simulink model "ExoskeletonControlModel"  (R2022b)
settings: Solver=ode3  StartTime=0.0  StopTime=inf  FixedStep=Ts  RelTol=1e-3
PreLoadFcn:
  | Ts_IO204 = 0.001;
  | 
  | if ~exist('Ts', 'var')
  | Ts = 0.001;
  | end
  | if ~exist('FPGA_Frequency', 'var')
  | FPGA_Frequency = 75000000;
  | end
  | 
  | ts_IO612 = 1e-3;
  | 
  | load('TargetReached.mat')
  | load('ActualPos_inc.mat')
model workspace (MAT data in the model file):
  DeltaData : timeseries (value not decoded)
  EC45_deg2incs = 2276
  EC60_deg2inc = 5461
  EC90_deg2incs = 7111
  Enc2rad_18bit = 2.3968e-05
  Enc2rad_19bit = 1.1984e-05
  Enc2rad_20bit = 5.9921e-06
  GiulioModel : robotics.RigidBodyTree (value not decoded)
  Giulio_Spheric_model : robotics.RigidBodyTree (value not decoded)
  Offset1_ticks = 571315
  Offset2_ticks = 590938.9928
  Offset3_ticks = 457912.8279
  Offset4_ticks = 482293.9763
  Offset5_ticks = 598735.9316
  Offset_M1 = 1.12645499896
  Offset_M2 = 4.02728553608
  Offset_M3 = 5.48587511336
  Offset_M4 = 2.03717511516
  Offset_M5 = 4.4996674016
  T1_Nm : object (value not decoded)
  T2_Nm : object (value not decoded)
  TBmodel : robotics.RigidBodyTree (value not decoded)
  Ts = 0.002
  Xg : object (value not decoded)
  Yg : object (value not decoded)
  Zg : object (value not decoded)
  a2 = 0.27
  change_variable = 0
  d1 = [0 0 0 0 0 0 0 0 0 0 0 0 ... (30001 elements, 30001x1)]
  d1_1 = 0.21074
  d2 = [0 0 0 0 0 0 0 0 0 0 0 0 ... (30001 elements, 30001x1)]
  d2_1 = 0.04864
  d3 = [0 0 0 0 0 0 0 0 0 0 0 0 ... (30001 elements, 30001x1)]
  d4 = [0 0 0 0 0 0 0 0 0 0 0 0 ... (30001 elements, 30001x1)]
  d5 = [0 0 0 0 0 0 0 0 0 0 0 0 ... (30001 elements, 30001x1)]
  d6 = [0 0 0 0 0 0 0 0 0 0 0 0 ... (30001 elements, 30001x1)]
  ee_x = -0.2852
  ee_y = -0.3683
  ee_z = -0.0386
  enc2rad_EC45 = 7.6699e-06
  enc2rad_EC90 = 2.3969e-05
  k1_Nm_ticks = 0.00923
  k2_Nm_ticks = 0.0257
  k3_Nm_ticks = 0.00692
  k4_Nm_ticks = 0.00729
  k5_Nm_ticks = 0.00641
  lower_lim_m1 = -330000
  lower_lim_m2 = -235302
  lower_lim_m3 = -132865
  lower_lim_m4 = -152732
  lower_lim_m5 = -138363
  lower_lim_m6 = -200325
  m1 = 2.441408578
  m2 = 3.750007
  m3 = 1.56250298
  m4 = 1.56250298
  m5 = 1.56250298
  m6 = 1.56250298
  n_oversampling = 8
  offset_sea_1 = 0.5547
  offset_sea_2 = 2.8595
  offset_sea_3 = 3.5058
  offset_sea_4 = 2.8586
  offset_sea_5 = 2.8736
  params : AKSIM (value not decoded)
  pos_th_neg = -180000
  pos_th_pos = 180000
  q1 = -1819347
  q2 = -196752
  q3 = -596465
  q4 = -556807
  q5 = -573932
  q6 = -489063
  sine = [0 0.187999937334 0.751998997352 1.69199492401 3.0079839574 4.6999608335 6.76791878442 9.21184953835 12.0317433196 15.2275888485 18.7993733417 22.7470825122 ... (12501 elements, 12501x1)]
  start : object (value not decoded)
  switch_admittance = 1
  t1 : object (value not decoded)
  t2 : object (value not decoded)
  torsionalStiffnes_M1 = 384.88
  torsionalStiffnes_M2 = 1500
  torsionalStiffnes_M3 = 901.97
  torsionalStiffnes_M4 = 950.86
  torsionalStiffnes_M5 = 930
  torsionalStiffnes_M6 = 914
  upper_lim_m1 = 340000
  upper_lim_m2 = 95467
  upper_lim_m3 = 164951
  upper_lim_m4 = 210607
  upper_lim_m5 = 252595
  upper_lim_m6 = 96694
  vel_th_neg = -100
  vel_th_pos = 100
  x = 0
undefined symbols (not defined in the file): C, DiscIntNeverNeededParam
libraries: canmsglib x285, speedgoatlib_IO614 x245, simulink x26, slrealtimeloglib x9, simulink_extras x6, robotmaniplib x6
(part 3 of 13)

== system ExoskeletonControlModel/DataProcessing/Working_Chart/GoHome.GoHome_M4.ST3_send_target_pos_M4 ==
  note: MOTOR 1 - TARGET POSITION
  Action Port : ActionPort
      settings: CopyFcn=Stateflow.SLINSF.SimulinkMan.removeBlockPreDeleteFcn  PreDeleteFcn=Stateflow.SLINSF.SimulinkMan.unsafePredeleteFcn
  receive_PDO3_m1 : Subsystem
  target_position_m1 : Constant  Value=0
  wires:
  target_position_m1/1 -> receive_PDO3_m1/1(target_pos)

== system ExoskeletonControlModel/DataProcessing/Working_Chart/GoHome.GoHome_M4.ST4_Abs_ref_start_immediatly_M4 ==
  note: MOTOR 1 - CONTROLWORD
  Action Port : ActionPort
      settings: CopyFcn=Stateflow.SLINSF.SimulinkMan.removeBlockPreDeleteFcn  PreDeleteFcn=Stateflow.SLINSF.SimulinkMan.unsafePredeleteFcn
  controlword_m1 : Constant  Value=63
  receive_PDO1_m1 : Subsystem
  wires:
  controlword_m1/1 -> receive_PDO1_m1/1(controlword)

== system ExoskeletonControlModel/DataProcessing/Working_Chart/GoHome.GoHome_M5.ST1_set_PPM_M5 ==
  note: MOTOR 1 - MODE & INTERPOLATION TIME PERIOD
  Action Port : ActionPort
      settings: CopyFcn=Stateflow.SLINSF.SimulinkMan.removeBlockPreDeleteFcn  PreDeleteFcn=Stateflow.SLINSF.SimulinkMan.unsafePredeleteFcn
  Bus Creator3 : BusCreator  Inputs=2
  interpolation_period_m1 : Constant  Value=10
  mode_m1 : Constant
  receive_PDO2_m1 : Subsystem
  wires:
  Bus Creator3/1 -> receive_PDO2_m1/1(mode)
  mode_m1/1 -> Bus Creator3/1  "mode_m1"
  interpolation_period_m1/1 -> Bus Creator3/2  "interpolation_period_m1"

== system ExoskeletonControlModel/DataProcessing/Working_Chart/GoHome.GoHome_M5.ST2_Switch_on_Enable_M5 ==
  note: MOTOR 1 - CONTROLWORD
  Action Port : ActionPort
      settings: CopyFcn=Stateflow.SLINSF.SimulinkMan.removeBlockPreDeleteFcn  PreDeleteFcn=Stateflow.SLINSF.SimulinkMan.unsafePredeleteFcn
  controlword_m1 : Constant  Value=15
  receive_PDO1_m1 : Subsystem
  wires:
  controlword_m1/1 -> receive_PDO1_m1/1(controlword)

== system ExoskeletonControlModel/DataProcessing/Working_Chart/GoHome.GoHome_M5.ST3_send_target_pos_M5 ==
  note: MOTOR 1 - TARGET POSITION
  Action Port : ActionPort
      settings: CopyFcn=Stateflow.SLINSF.SimulinkMan.removeBlockPreDeleteFcn  PreDeleteFcn=Stateflow.SLINSF.SimulinkMan.unsafePredeleteFcn
  receive_PDO3_m1 : Subsystem
  target_position_m1 : Constant  Value=0
  wires:
  target_position_m1/1 -> receive_PDO3_m1/1(target_pos)

== system ExoskeletonControlModel/DataProcessing/Working_Chart/GoHome.GoHome_M5.ST4_Abs_ref_start_immediatly_M5 ==
  note: MOTOR 1 - CONTROLWORD
  Action Port : ActionPort
      settings: CopyFcn=Stateflow.SLINSF.SimulinkMan.removeBlockPreDeleteFcn  PreDeleteFcn=Stateflow.SLINSF.SimulinkMan.unsafePredeleteFcn
  controlword_m1 : Constant  Value=63
  receive_PDO1_m1 : Subsystem
  wires:
  controlword_m1/1 -> receive_PDO1_m1/1(controlword)

== system ExoskeletonControlModel/DataProcessing/Working_Chart/GoHome.GoHome_M6.ST1_set_PPM_M6 ==
  note: MOTOR 1 - MODE & INTERPOLATION TIME PERIOD
  Action Port : ActionPort
      settings: CopyFcn=Stateflow.SLINSF.SimulinkMan.removeBlockPreDeleteFcn  PreDeleteFcn=Stateflow.SLINSF.SimulinkMan.unsafePredeleteFcn
  Bus Creator3 : BusCreator  Inputs=2
  interpolation_period_m1 : Constant  Value=10
  mode_m1 : Constant
  receive_PDO2_m1 : Subsystem
  wires:
  Bus Creator3/1 -> receive_PDO2_m1/1(mode)
  mode_m1/1 -> Bus Creator3/1  "mode_m1"
  interpolation_period_m1/1 -> Bus Creator3/2  "interpolation_period_m1"

== system ExoskeletonControlModel/DataProcessing/Working_Chart/GoHome.GoHome_M6.ST2_Switch_on_Enable_M6 ==
  note: MOTOR 1 - CONTROLWORD
  Action Port : ActionPort
      settings: CopyFcn=Stateflow.SLINSF.SimulinkMan.removeBlockPreDeleteFcn  PreDeleteFcn=Stateflow.SLINSF.SimulinkMan.unsafePredeleteFcn
  controlword_m1 : Constant  Value=15
  receive_PDO1_m1 : Subsystem
  wires:
  controlword_m1/1 -> receive_PDO1_m1/1(controlword)

== system ExoskeletonControlModel/DataProcessing/Working_Chart/GoHome.GoHome_M6.ST3_send_target_pos_M6 ==
  note: MOTOR 1 - TARGET POSITION
  Action Port : ActionPort
      settings: CopyFcn=Stateflow.SLINSF.SimulinkMan.removeBlockPreDeleteFcn  PreDeleteFcn=Stateflow.SLINSF.SimulinkMan.unsafePredeleteFcn
  receive_PDO3_m1 : Subsystem
  target_position_m1 : Constant  Value=0
  wires:
  target_position_m1/1 -> receive_PDO3_m1/1(target_pos)

== system ExoskeletonControlModel/DataProcessing/Working_Chart/GoHome.GoHome_M6.ST4_Abs_ref_start_immediatly_M6 ==
  note: MOTOR 1 - CONTROLWORD
  Action Port : ActionPort
      settings: CopyFcn=Stateflow.SLINSF.SimulinkMan.removeBlockPreDeleteFcn  PreDeleteFcn=Stateflow.SLINSF.SimulinkMan.unsafePredeleteFcn
  controlword_m1 : Constant  Value=63
  receive_PDO1_m1 : Subsystem
  wires:
  controlword_m1/1 -> receive_PDO1_m1/1(controlword)

== system ExoskeletonControlModel/DataProcessing/Working_Chart/Transparency.Block_not_recorded_joints.ST1_set_CSP_M1 ==
  note: MOTOR 1 - MODE & INTERPOLATION TIME PERIOD
  Action Port : ActionPort
      settings: CopyFcn=Stateflow.SLINSF.SimulinkMan.removeBlockPreDeleteFcn  PreDeleteFcn=Stateflow.SLINSF.SimulinkMan.unsafePredeleteFcn
  Bus Creator3 : BusCreator  Inputs=2
  interpolation_period_m1 : Constant  Value=20
  mode_m1 : Constant  Value=8
  receive_PDO2_m1 : Subsystem
  wires:
  Bus Creator3/1 -> receive_PDO2_m1/1(mode)
  mode_m1/1 -> Bus Creator3/1  "mode_m1"
  interpolation_period_m1/1 -> Bus Creator3/2  "interpolation_period_m1"

== system ExoskeletonControlModel/DataProcessing/Working_Chart/Transparency.Block_not_recorded_joints.ST1_set_CSP_M6 ==
  note: MOTOR 1 - MODE & INTERPOLATION TIME PERIOD
  Action Port : ActionPort
      settings: CopyFcn=Stateflow.SLINSF.SimulinkMan.removeBlockPreDeleteFcn  PreDeleteFcn=Stateflow.SLINSF.SimulinkMan.unsafePredeleteFcn
  Bus Creator3 : BusCreator  Inputs=2
  interpolation_period_m1 : Constant  Value=20
  mode_m1 : Constant  Value=8
  receive_PDO2_m1 : Subsystem
  wires:
  Bus Creator3/1 -> receive_PDO2_m1/1(mode)
  mode_m1/1 -> Bus Creator3/1  "mode_m1"
  interpolation_period_m1/1 -> Bus Creator3/2  "interpolation_period_m1"

== system ExoskeletonControlModel/DataProcessing/Working_Chart/Transparency.GoToExerciseHome.GoHome_M1.ST1_set_PPM_M1 ==
  note: MOTOR 1 - MODE & INTERPOLATION TIME PERIOD
  Action Port : ActionPort
      settings: CopyFcn=Stateflow.SLINSF.SimulinkMan.removeBlockPreDeleteFcn  PreDeleteFcn=Stateflow.SLINSF.SimulinkMan.unsafePredeleteFcn
  Bus Creator3 : BusCreator  Inputs=2
  interpolation_period_m1 : Constant  Value=10
  mode_m1 : Constant
  receive_PDO2_m1 : Subsystem
  wires:
  Bus Creator3/1 -> receive_PDO2_m1/1(mode)
  mode_m1/1 -> Bus Creator3/1  "mode_m1"
  interpolation_period_m1/1 -> Bus Creator3/2  "interpolation_period_m1"

== system ExoskeletonControlModel/DataProcessing/Working_Chart/Transparency.GoToExerciseHome.GoHome_M1.ST2_Switch_on_Enable_M1 ==
  note: MOTOR 1 - CONTROLWORD
  Action Port : ActionPort
      settings: CopyFcn=Stateflow.SLINSF.SimulinkMan.removeBlockPreDeleteFcn  PreDeleteFcn=Stateflow.SLINSF.SimulinkMan.unsafePredeleteFcn
  controlword_m1 : Constant  Value=15
  receive_PDO1_m1 : Subsystem
  wires:
  controlword_m1/1 -> receive_PDO1_m1/1(controlword)

== system ExoskeletonControlModel/DataProcessing/Working_Chart/Transparency.GoToExerciseHome.GoHome_M1.ST3_send_target_pos_M1 ==
  note: MOTOR 1 - TARGET POSITION
  Action Port : ActionPort
      settings: CopyFcn=Stateflow.SLINSF.SimulinkMan.removeBlockPreDeleteFcn  PreDeleteFcn=Stateflow.SLINSF.SimulinkMan.unsafePredeleteFcn
  receive_PDO3_m1 : Subsystem
  target_position_m1 : Constant  Value=0
  wires:
  target_position_m1/1 -> receive_PDO3_m1/1(target_pos)

== system ExoskeletonControlModel/DataProcessing/Working_Chart/Transparency.GoToExerciseHome.GoHome_M1.ST4_Abs_ref_start_immediatly_M1 ==
  note: MOTOR 1 - CONTROLWORD
  Action Port : ActionPort
      settings: CopyFcn=Stateflow.SLINSF.SimulinkMan.removeBlockPreDeleteFcn  PreDeleteFcn=Stateflow.SLINSF.SimulinkMan.unsafePredeleteFcn
  controlword_m1 : Constant  Value=63
  receive_PDO1_m1 : Subsystem
  wires:
  controlword_m1/1 -> receive_PDO1_m1/1(controlword)

== system ExoskeletonControlModel/DataProcessing/Working_Chart/Transparency.GoToExerciseHome.GoHome_M2.ST1_set_PPM_M2 ==
  note: MOTOR 1 - MODE & INTERPOLATION TIME PERIOD
  Action Port : ActionPort
      settings: CopyFcn=Stateflow.SLINSF.SimulinkMan.removeBlockPreDeleteFcn  PreDeleteFcn=Stateflow.SLINSF.SimulinkMan.unsafePredeleteFcn
  Bus Creator3 : BusCreator  Inputs=2
  interpolation_period_m1 : Constant  Value=10
  mode_m1 : Constant
  receive_PDO2_m1 : Subsystem
  wires:
  Bus Creator3/1 -> receive_PDO2_m1/1(mode)
  mode_m1/1 -> Bus Creator3/1  "mode_m1"
  interpolation_period_m1/1 -> Bus Creator3/2  "interpolation_period_m1"

== system ExoskeletonControlModel/DataProcessing/Working_Chart/Transparency.GoToExerciseHome.GoHome_M2.ST2_Switch_on_Enable_M2 ==
  note: MOTOR 1 - CONTROLWORD
  Action Port : ActionPort
      settings: CopyFcn=Stateflow.SLINSF.SimulinkMan.removeBlockPreDeleteFcn  PreDeleteFcn=Stateflow.SLINSF.SimulinkMan.unsafePredeleteFcn
  controlword_m1 : Constant  Value=15
  receive_PDO1_m1 : Subsystem
  wires:
  controlword_m1/1 -> receive_PDO1_m1/1(controlword)

== system ExoskeletonControlModel/DataProcessing/Working_Chart/Transparency.GoToExerciseHome.GoHome_M2.ST3_send_target_pos_M2 ==
  note: MOTOR 1 - TARGET POSITION
  Action Port : ActionPort
      settings: CopyFcn=Stateflow.SLINSF.SimulinkMan.removeBlockPreDeleteFcn  PreDeleteFcn=Stateflow.SLINSF.SimulinkMan.unsafePredeleteFcn
  receive_PDO3_m1 : Subsystem
  target_position_m1 : Constant  Value=0
  wires:
  target_position_m1/1 -> receive_PDO3_m1/1(target_pos)

== system ExoskeletonControlModel/DataProcessing/Working_Chart/Transparency.GoToExerciseHome.GoHome_M2.ST4_Abs_ref_start_immediatly_M2 ==
  note: MOTOR 1 - CONTROLWORD
  Action Port : ActionPort
      settings: CopyFcn=Stateflow.SLINSF.SimulinkMan.removeBlockPreDeleteFcn  PreDeleteFcn=Stateflow.SLINSF.SimulinkMan.unsafePredeleteFcn
  controlword_m1 : Constant  Value=63
  receive_PDO1_m1 : Subsystem
  wires:
  controlword_m1/1 -> receive_PDO1_m1/1(controlword)

== system ExoskeletonControlModel/DataProcessing/Working_Chart/Transparency.GoToExerciseHome.GoHome_M3.ST1_set_PPM_M3 ==
  note: MOTOR 1 - MODE & INTERPOLATION TIME PERIOD
  Action Port : ActionPort
      settings: CopyFcn=Stateflow.SLINSF.SimulinkMan.removeBlockPreDeleteFcn  PreDeleteFcn=Stateflow.SLINSF.SimulinkMan.unsafePredeleteFcn
  Bus Creator3 : BusCreator  Inputs=2
  interpolation_period_m1 : Constant  Value=10
  mode_m1 : Constant
  receive_PDO2_m1 : Subsystem
  wires:
  Bus Creator3/1 -> receive_PDO2_m1/1(mode)
  mode_m1/1 -> Bus Creator3/1  "mode_m1"
  interpolation_period_m1/1 -> Bus Creator3/2  "interpolation_period_m1"

== system ExoskeletonControlModel/DataProcessing/Working_Chart/Transparency.GoToExerciseHome.GoHome_M3.ST2_Switch_on_Enable_M3 ==
  note: MOTOR 1 - CONTROLWORD
  Action Port : ActionPort
      settings: CopyFcn=Stateflow.SLINSF.SimulinkMan.removeBlockPreDeleteFcn  PreDeleteFcn=Stateflow.SLINSF.SimulinkMan.unsafePredeleteFcn
  controlword_m1 : Constant  Value=15
  receive_PDO1_m1 : Subsystem
  wires:
  controlword_m1/1 -> receive_PDO1_m1/1(controlword)

== system ExoskeletonControlModel/DataProcessing/Working_Chart/Transparency.GoToExerciseHome.GoHome_M3.ST3_send_target_pos_M3 ==
  note: MOTOR 3 - TARGET POSITION
  Action Port : ActionPort
      settings: CopyFcn=Stateflow.SLINSF.SimulinkMan.removeBlockPreDeleteFcn  PreDeleteFcn=Stateflow.SLINSF.SimulinkMan.unsafePredeleteFcn
  receive_PDO3_m1 : Subsystem
  target_position_m1 : Constant  Value=50153
  wires:
  target_position_m1/1 -> receive_PDO3_m1/1(target_pos)

== system ExoskeletonControlModel/DataProcessing/Working_Chart/Transparency.GoToExerciseHome.GoHome_M3.ST4_Abs_ref_start_immediatly_M3 ==
  note: MOTOR 1 - CONTROLWORD
  Action Port : ActionPort
      settings: CopyFcn=Stateflow.SLINSF.SimulinkMan.removeBlockPreDeleteFcn  PreDeleteFcn=Stateflow.SLINSF.SimulinkMan.unsafePredeleteFcn
  controlword_m1 : Constant  Value=63
  receive_PDO1_m1 : Subsystem
  wires:
  controlword_m1/1 -> receive_PDO1_m1/1(controlword)

== system ExoskeletonControlModel/DataProcessing/Working_Chart/Transparency.GoToExerciseHome.GoHome_M4.ST1_set_PPM_M4 ==
  note: MOTOR 1 - MODE & INTERPOLATION TIME PERIOD
  Action Port : ActionPort
      settings: CopyFcn=Stateflow.SLINSF.SimulinkMan.removeBlockPreDeleteFcn  PreDeleteFcn=Stateflow.SLINSF.SimulinkMan.unsafePredeleteFcn
  Bus Creator3 : BusCreator  Inputs=2
  interpolation_period_m1 : Constant  Value=10
  mode_m1 : Constant
  receive_PDO2_m1 : Subsystem
  wires:
  Bus Creator3/1 -> receive_PDO2_m1/1(mode)
  mode_m1/1 -> Bus Creator3/1  "mode_m1"
  interpolation_period_m1/1 -> Bus Creator3/2  "interpolation_period_m1"

== system ExoskeletonControlModel/DataProcessing/Working_Chart/Transparency.GoToExerciseHome.GoHome_M4.ST2_Switch_on_Enable_M4 ==
  note: MOTOR 1 - CONTROLWORD
  Action Port : ActionPort
      settings: CopyFcn=Stateflow.SLINSF.SimulinkMan.removeBlockPreDeleteFcn  PreDeleteFcn=Stateflow.SLINSF.SimulinkMan.unsafePredeleteFcn
  controlword_m1 : Constant  Value=15
  receive_PDO1_m1 : Subsystem
  wires:
  controlword_m1/1 -> receive_PDO1_m1/1(controlword)

== system ExoskeletonControlModel/DataProcessing/Working_Chart/Transparency.GoToExerciseHome.GoHome_M4.ST3_send_target_pos_M4 ==
  note: MOTOR 4 - TARGET POSITION
  Action Port : ActionPort
      settings: CopyFcn=Stateflow.SLINSF.SimulinkMan.removeBlockPreDeleteFcn  PreDeleteFcn=Stateflow.SLINSF.SimulinkMan.unsafePredeleteFcn
  receive_PDO3_m1 : Subsystem
  target_position_m1 : Constant  Value=-22699
  wires:
  target_position_m1/1 -> receive_PDO3_m1/1(target_pos)

== system ExoskeletonControlModel/DataProcessing/Working_Chart/Transparency.GoToExerciseHome.GoHome_M4.ST3_send_target_pos_M4_abd ==
  note: MOTOR 4 - TARGET POSITION
  Action Port : ActionPort
      settings: CopyFcn=Stateflow.SLINSF.SimulinkMan.removeBlockPreDeleteFcn  PreDeleteFcn=Stateflow.SLINSF.SimulinkMan.unsafePredeleteFcn
  receive_PDO3_m1 : Subsystem
  target_position_m1 : Constant  Value=-90979
  wires:
  target_position_m1/1 -> receive_PDO3_m1/1(target_pos)

== system ExoskeletonControlModel/DataProcessing/Working_Chart/Transparency.GoToExerciseHome.GoHome_M4.ST4_Abs_ref_start_immediatly_M4 ==
  note: MOTOR 1 - CONTROLWORD
  Action Port : ActionPort
      settings: CopyFcn=Stateflow.SLINSF.SimulinkMan.removeBlockPreDeleteFcn  PreDeleteFcn=Stateflow.SLINSF.SimulinkMan.unsafePredeleteFcn
  controlword_m1 : Constant  Value=63
  receive_PDO1_m1 : Subsystem
  wires:
  controlword_m1/1 -> receive_PDO1_m1/1(controlword)

== system ExoskeletonControlModel/DataProcessing/Working_Chart/Transparency.GoToExerciseHome.GoHome_M5.ST1_set_PPM_M5 ==
  note: MOTOR 1 - MODE & INTERPOLATION TIME PERIOD
  Action Port : ActionPort
      settings: CopyFcn=Stateflow.SLINSF.SimulinkMan.removeBlockPreDeleteFcn  PreDeleteFcn=Stateflow.SLINSF.SimulinkMan.unsafePredeleteFcn
  Bus Creator3 : BusCreator  Inputs=2
  interpolation_period_m1 : Constant  Value=10
  mode_m1 : Constant
  receive_PDO2_m1 : Subsystem
  wires:
  Bus Creator3/1 -> receive_PDO2_m1/1(mode)
  mode_m1/1 -> Bus Creator3/1  "mode_m1"
  interpolation_period_m1/1 -> Bus Creator3/2  "interpolation_period_m1"

== system ExoskeletonControlModel/DataProcessing/Working_Chart/Transparency.GoToExerciseHome.GoHome_M5.ST2_Switch_on_Enable_M5 ==
  note: MOTOR 1 - CONTROLWORD
  Action Port : ActionPort
      settings: CopyFcn=Stateflow.SLINSF.SimulinkMan.removeBlockPreDeleteFcn  PreDeleteFcn=Stateflow.SLINSF.SimulinkMan.unsafePredeleteFcn
  controlword_m1 : Constant  Value=15
  receive_PDO1_m1 : Subsystem
  wires:
  controlword_m1/1 -> receive_PDO1_m1/1(controlword)

== system ExoskeletonControlModel/DataProcessing/Working_Chart/Transparency.GoToExerciseHome.GoHome_M5.ST3_send_target_pos_M5 ==
  note: MOTOR 5 - TARGET POSITION
  Action Port : ActionPort
      settings: CopyFcn=Stateflow.SLINSF.SimulinkMan.removeBlockPreDeleteFcn  PreDeleteFcn=Stateflow.SLINSF.SimulinkMan.unsafePredeleteFcn
  receive_PDO3_m1 : Subsystem
  target_position_m1 : Constant  Value=-9784
  wires:
  target_position_m1/1 -> receive_PDO3_m1/1(target_pos)

== system ExoskeletonControlModel/DataProcessing/Working_Chart/Transparency.GoToExerciseHome.GoHome_M5.ST4_Abs_ref_start_immediatly_M5 ==
  note: MOTOR 1 - CONTROLWORD
  Action Port : ActionPort
      settings: CopyFcn=Stateflow.SLINSF.SimulinkMan.removeBlockPreDeleteFcn  PreDeleteFcn=Stateflow.SLINSF.SimulinkMan.unsafePredeleteFcn
  controlword_m1 : Constant  Value=63
  receive_PDO1_m1 : Subsystem
  wires:
  controlword_m1/1 -> receive_PDO1_m1/1(controlword)

== system ExoskeletonControlModel/DataProcessing/Working_Chart/Transparency.GoToExerciseHome.GoHome_M6.ST1_set_PPM_M6 ==
  note: MOTOR 1 - MODE & INTERPOLATION TIME PERIOD
  Action Port : ActionPort
      settings: CopyFcn=Stateflow.SLINSF.SimulinkMan.removeBlockPreDeleteFcn  PreDeleteFcn=Stateflow.SLINSF.SimulinkMan.unsafePredeleteFcn
  Bus Creator3 : BusCreator  Inputs=2
  interpolation_period_m1 : Constant  Value=10
  mode_m1 : Constant
  receive_PDO2_m1 : Subsystem
  wires:
  Bus Creator3/1 -> receive_PDO2_m1/1(mode)
  mode_m1/1 -> Bus Creator3/1  "mode_m1"
  interpolation_period_m1/1 -> Bus Creator3/2  "interpolation_period_m1"

== system ExoskeletonControlModel/DataProcessing/Working_Chart/Transparency.GoToExerciseHome.GoHome_M6.ST2_Switch_on_Enable_M6 ==
  note: MOTOR 1 - CONTROLWORD
  Action Port : ActionPort
      settings: CopyFcn=Stateflow.SLINSF.SimulinkMan.removeBlockPreDeleteFcn  PreDeleteFcn=Stateflow.SLINSF.SimulinkMan.unsafePredeleteFcn
  controlword_m1 : Constant  Value=15
  receive_PDO1_m1 : Subsystem
  wires:
  controlword_m1/1 -> receive_PDO1_m1/1(controlword)

== system ExoskeletonControlModel/DataProcessing/Working_Chart/Transparency.GoToExerciseHome.GoHome_M6.ST3_send_target_pos_M6 ==
  note: MOTOR 1 - TARGET POSITION
  Action Port : ActionPort
      settings: CopyFcn=Stateflow.SLINSF.SimulinkMan.removeBlockPreDeleteFcn  PreDeleteFcn=Stateflow.SLINSF.SimulinkMan.unsafePredeleteFcn
  receive_PDO3_m1 : Subsystem
  target_position_m1 : Constant  Value=-165590
  wires:
  target_position_m1/1 -> receive_PDO3_m1/1(target_pos)

== system ExoskeletonControlModel/DataProcessing/Working_Chart/Transparency.GoToExerciseHome.GoHome_M6.ST4_Abs_ref_start_immediatly_M6 ==
  note: MOTOR 1 - CONTROLWORD
  Action Port : ActionPort
      settings: CopyFcn=Stateflow.SLINSF.SimulinkMan.removeBlockPreDeleteFcn  PreDeleteFcn=Stateflow.SLINSF.SimulinkMan.unsafePredeleteFcn
  controlword_m1 : Constant  Value=63
  receive_PDO1_m1 : Subsystem
  wires:
  controlword_m1/1 -> receive_PDO1_m1/1(controlword)

== system ExoskeletonControlModel/DataProcessing/Working_Chart/Transparency.ImpedanceMode.ShoulderFlexion.ST1_set_CSP_M3 ==
  note: MOTOR 1 - MODE & INTERPOLATION TIME PERIOD
  Action Port : ActionPort
      settings: CopyFcn=Stateflow.SLINSF.SimulinkMan.removeBlockPreDeleteFcn  PreDeleteFcn=Stateflow.SLINSF.SimulinkMan.unsafePredeleteFcn
  Bus Creator3 : BusCreator  Inputs=2
  interpolation_period_m1 : Constant  Value=10
  mode_m1 : Constant  Value=8
  receive_PDO2_m1 : Subsystem
  wires:
  Bus Creator3/1 -> receive_PDO2_m1/1(mode)
  mode_m1/1 -> Bus Creator3/1  "mode_m1"
  interpolation_period_m1/1 -> Bus Creator3/2  "interpolation_period_m1"

== system ExoskeletonControlModel/DataProcessing/Working_Chart/Transparency.ImpedanceMode.ShoulderFlexion.ST1_set_CSP_M4 ==
  note: MOTOR 1 - MODE & INTERPOLATION TIME PERIOD
  Action Port : ActionPort
      settings: CopyFcn=Stateflow.SLINSF.SimulinkMan.removeBlockPreDeleteFcn  PreDeleteFcn=Stateflow.SLINSF.SimulinkMan.unsafePredeleteFcn
  Bus Creator3 : BusCreator  Inputs=2
  interpolation_period_m1 : Constant  Value=10
  mode_m1 : Constant  Value=8
  receive_PDO2_m1 : Subsystem
  wires:
  Bus Creator3/1 -> receive_PDO2_m1/1(mode)
  mode_m1/1 -> Bus Creator3/1  "mode_m1"
  interpolation_period_m1/1 -> Bus Creator3/2  "interpolation_period_m1"

== system ExoskeletonControlModel/DataProcessing/Working_Chart/Transparency.ImpedanceMode.ShoulderFlexion.ST1_set_CSP_M6 ==
  note: MOTOR 1 - MODE & INTERPOLATION TIME PERIOD
  Action Port : ActionPort
      settings: CopyFcn=Stateflow.SLINSF.SimulinkMan.removeBlockPreDeleteFcn  PreDeleteFcn=Stateflow.SLINSF.SimulinkMan.unsafePredeleteFcn
  Bus Creator3 : BusCreator  Inputs=2
  interpolation_period_m1 : Constant  Value=10
  mode_m1 : Constant  Value=8
  receive_PDO2_m1 : Subsystem
  wires:
  Bus Creator3/1 -> receive_PDO2_m1/1(mode)
  mode_m1/1 -> Bus Creator3/1  "mode_m1"
  interpolation_period_m1/1 -> Bus Creator3/2  "interpolation_period_m1"

== system ExoskeletonControlModel/DataProcessing/Working_Chart/Transparency.ResetState ==
  Action Port : ActionPort
      settings: CopyFcn=Stateflow.SLINSF.SimulinkMan.removeBlockPreDeleteFcn  PreDeleteFcn=Stateflow.SLINSF.SimulinkMan.unsafePredeleteFcn
  Constant{,1..17} (18 alike) : Constant  Value=0
  Data Store Write : DataStoreWrite  DataStoreName=Start_m1  IndexOptions=Index vector (dialog)  Indices=1  OutputSizes=1
  Data Store Write1 : DataStoreWrite  DataStoreName=Start_m3  IndexOptions=Index vector (dialog)  Indices=1  OutputSizes=1
  Data Store Write10 : DataStoreWrite  DataStoreName=Spring_m5  IndexOptions=Index vector (dialog)  Indices=1  OutputSizes=1
  Data Store Write11 : DataStoreWrite  DataStoreName=Spring_m6  IndexOptions=Index vector (dialog)  Indices=1  OutputSizes=1
  Data Store Write12 : DataStoreWrite  DataStoreName=Damper_m5  IndexOptions=Index vector (dialog)  Indices=1  OutputSizes=1
  Data Store Write13 : DataStoreWrite  DataStoreName=Damper_m6  IndexOptions=Index vector (dialog)  Indices=1  OutputSizes=1
  Data Store Write14 : DataStoreWrite  DataStoreName=Damper_m1  IndexOptions=Index vector (dialog)  Indices=1  OutputSizes=1
  Data Store Write15 : DataStoreWrite  DataStoreName=Damper_m3  IndexOptions=Index vector (dialog)  Indices=1  OutputSizes=1
  Data Store Write16 : DataStoreWrite  DataStoreName=Damper_m2  IndexOptions=Index vector (dialog)  Indices=1  OutputSizes=1
  Data Store Write17 : DataStoreWrite  DataStoreName=Damper_m4  IndexOptions=Index vector (dialog)  Indices=1  OutputSizes=1
  Data Store Write2 : DataStoreWrite  DataStoreName=Start_m2  IndexOptions=Index vector (dialog)  Indices=1  OutputSizes=1
  Data Store Write3 : DataStoreWrite  DataStoreName=Start_m4  IndexOptions=Index vector (dialog)  Indices=1  OutputSizes=1
  Data Store Write4 : DataStoreWrite  DataStoreName=Start_m5  IndexOptions=Index vector (dialog)  Indices=1  OutputSizes=1
  Data Store Write5 : DataStoreWrite  DataStoreName=Start_m6  IndexOptions=Index vector (dialog)  Indices=1  OutputSizes=1
  Data Store Write6 : DataStoreWrite  DataStoreName=Spring_m1  IndexOptions=Index vector (dialog)  Indices=1  OutputSizes=1
  Data Store Write7 : DataStoreWrite  DataStoreName=Spring_m3  IndexOptions=Index vector (dialog)  Indices=1  OutputSizes=1
  Data Store Write8 : DataStoreWrite  DataStoreName=Spring_m2  IndexOptions=Index vector (dialog)  Indices=1  OutputSizes=1
  Data Store Write9 : DataStoreWrite  DataStoreName=Spring_m4  IndexOptions=Index vector (dialog)  Indices=1  OutputSizes=1
  wires:
  Constant/1 -> Data Store Write/1
  Constant1/1 -> Data Store Write1/1
  Constant2/1 -> Data Store Write2/1
  Constant3/1 -> Data Store Write3/1
  Constant4/1 -> Data Store Write4/1
  Constant5/1 -> Data Store Write5/1
  Constant6/1 -> Data Store Write6/1
  Constant11/1 -> Data Store Write11/1
  Constant8/1 -> Data Store Write8/1
  Constant7/1 -> Data Store Write7/1
  Constant9/1 -> Data Store Write9/1
  Constant10/1 -> Data Store Write10/1
  Constant17/1 -> Data Store Write17/1
  Constant13/1 -> Data Store Write13/1
  Constant12/1 -> Data Store Write12/1
  Constant14/1 -> Data Store Write14/1
  Constant16/1 -> Data Store Write16/1
  Constant15/1 -> Data Store Write15/1

== system ExoskeletonControlModel/DataProcessing/Working_Chart/Transparency.SET_MODE.ST1_set_CSP_M2 ==
  note: MOTOR 1 - MODE & INTERPOLATION TIME PERIOD
  Action Port : ActionPort
      settings: CopyFcn=Stateflow.SLINSF.SimulinkMan.removeBlockPreDeleteFcn  PreDeleteFcn=Stateflow.SLINSF.SimulinkMan.unsafePredeleteFcn
  Bus Creator3 : BusCreator  Inputs=2
  interpolation_period_m1 : Constant  Value=10
  mode_m1 : Constant  Value=8
  receive_PDO2_m1 : Subsystem
  wires:
  Bus Creator3/1 -> receive_PDO2_m1/1(mode)
  mode_m1/1 -> Bus Creator3/1  "mode_m1"
  interpolation_period_m1/1 -> Bus Creator3/2  "interpolation_period_m1"

== system ExoskeletonControlModel/DataProcessing/Working_Chart/Transparency.SET_MODE.ST1_set_CST_M1 ==
  note: MOTOR 1 - MODE & INTERPOLATION TIME PERIOD
  Action Port : ActionPort
      settings: CopyFcn=Stateflow.SLINSF.SimulinkMan.removeBlockPreDeleteFcn  PreDeleteFcn=Stateflow.SLINSF.SimulinkMan.unsafePredeleteFcn
  Bus Creator3 : BusCreator  Inputs=2
  interpolation_period_m1 : Constant  Value=20
  mode_m1 : Constant  Value=10
  receive_PDO2_m1 : Subsystem
  wires:
  Bus Creator3/1 -> receive_PDO2_m1/1(mode)
  mode_m1/1 -> Bus Creator3/1  "mode_m1"
  interpolation_period_m1/1 -> Bus Creator3/2  "interpolation_period_m1"

== system ExoskeletonControlModel/DataProcessing/Working_Chart/Transparency.SET_MODE.ST1_set_CST_M3 ==
  note: MOTOR 1 - MODE & INTERPOLATION TIME PERIOD
  Action Port : ActionPort
      settings: CopyFcn=Stateflow.SLINSF.SimulinkMan.removeBlockPreDeleteFcn  PreDeleteFcn=Stateflow.SLINSF.SimulinkMan.unsafePredeleteFcn
  Bus Creator3 : BusCreator  Inputs=2
  interpolation_period_m1 : Constant  Value=10
  mode_m1 : Constant  Value=10
  receive_PDO2_m1 : Subsystem
  wires:
  Bus Creator3/1 -> receive_PDO2_m1/1(mode)
  mode_m1/1 -> Bus Creator3/1  "mode_m1"
  interpolation_period_m1/1 -> Bus Creator3/2  "interpolation_period_m1"

== system ExoskeletonControlModel/DataProcessing/Working_Chart/Transparency.SET_MODE.ST1_set_CST_M4 ==
  note: MOTOR 1 - MODE & INTERPOLATION TIME PERIOD
  Action Port : ActionPort
      settings: CopyFcn=Stateflow.SLINSF.SimulinkMan.removeBlockPreDeleteFcn  PreDeleteFcn=Stateflow.SLINSF.SimulinkMan.unsafePredeleteFcn
  Bus Creator3 : BusCreator  Inputs=2
  interpolation_period_m1 : Constant  Value=10
  mode_m1 : Constant  Value=10
  receive_PDO2_m1 : Subsystem
  wires:
  Bus Creator3/1 -> receive_PDO2_m1/1(mode)
  mode_m1/1 -> Bus Creator3/1  "mode_m1"
  interpolation_period_m1/1 -> Bus Creator3/2  "interpolation_period_m1"

== system ExoskeletonControlModel/DataProcessing/Working_Chart/Transparency.SET_MODE.ST1_set_CST_M5 ==
  note: MOTOR 1 - MODE & INTERPOLATION TIME PERIOD
  Action Port : ActionPort
      settings: CopyFcn=Stateflow.SLINSF.SimulinkMan.removeBlockPreDeleteFcn  PreDeleteFcn=Stateflow.SLINSF.SimulinkMan.unsafePredeleteFcn
  Bus Creator3 : BusCreator  Inputs=2
  interpolation_period_m1 : Constant  Value=20
  mode_m1 : Constant  Value=10
  receive_PDO2_m1 : Subsystem
  wires:
  Bus Creator3/1 -> receive_PDO2_m1/1(mode)
  mode_m1/1 -> Bus Creator3/1  "mode_m1"
  interpolation_period_m1/1 -> Bus Creator3/2  "interpolation_period_m1"

== system ExoskeletonControlModel/DataProcessing/Working_Chart/Transparency.SET_MODE.ST1_set_CST_M6 ==
  note: MOTOR 1 - MODE & INTERPOLATION TIME PERIOD
  Action Port : ActionPort
      settings: CopyFcn=Stateflow.SLINSF.SimulinkMan.removeBlockPreDeleteFcn  PreDeleteFcn=Stateflow.SLINSF.SimulinkMan.unsafePredeleteFcn
  Bus Creator3 : BusCreator  Inputs=2
  interpolation_period_m1 : Constant  Value=20
  mode_m1 : Constant  Value=10
  receive_PDO2_m1 : Subsystem
  wires:
  Bus Creator3/1 -> receive_PDO2_m1/1(mode)
  mode_m1/1 -> Bus Creator3/1  "mode_m1"
  interpolation_period_m1/1 -> Bus Creator3/2  "interpolation_period_m1"

== system ExoskeletonControlModel/DataProcessing/Working_Chart/Transparency.SetCSPforALL.ST1_set_CSP_M1 ==
  note: MOTOR 1 - MODE & INTERPOLATION TIME PERIOD
  Action Port : ActionPort
      settings: CopyFcn=Stateflow.SLINSF.SimulinkMan.removeBlockPreDeleteFcn  PreDeleteFcn=Stateflow.SLINSF.SimulinkMan.unsafePredeleteFcn
  Bus Creator3 : BusCreator  Inputs=2
  interpolation_period_m1 : Constant  Value=10
  mode_m1 : Constant  Value=8
  receive_PDO2_m1 : Subsystem
  wires:
  Bus Creator3/1 -> receive_PDO2_m1/1(mode)
  mode_m1/1 -> Bus Creator3/1  "mode_m1"
  interpolation_period_m1/1 -> Bus Creator3/2  "interpolation_period_m1"

== system ExoskeletonControlModel/DataProcessing/Working_Chart/Transparency.SetCSPforALL.ST1_set_CSP_M2 ==
  note: MOTOR 1 - MODE & INTERPOLATION TIME PERIOD
  Action Port : ActionPort
      settings: CopyFcn=Stateflow.SLINSF.SimulinkMan.removeBlockPreDeleteFcn  PreDeleteFcn=Stateflow.SLINSF.SimulinkMan.unsafePredeleteFcn
  Bus Creator3 : BusCreator  Inputs=2
  interpolation_period_m1 : Constant  Value=10
  mode_m1 : Constant  Value=8
  receive_PDO2_m1 : Subsystem
  wires:
  Bus Creator3/1 -> receive_PDO2_m1/1(mode)
  mode_m1/1 -> Bus Creator3/1  "mode_m1"
  interpolation_period_m1/1 -> Bus Creator3/2  "interpolation_period_m1"

== system ExoskeletonControlModel/DataProcessing/Working_Chart/Transparency.SetCSPforALL.ST1_set_CSP_M3 ==
  note: MOTOR 1 - MODE & INTERPOLATION TIME PERIOD
  Action Port : ActionPort
      settings: CopyFcn=Stateflow.SLINSF.SimulinkMan.removeBlockPreDeleteFcn  PreDeleteFcn=Stateflow.SLINSF.SimulinkMan.unsafePredeleteFcn
  Bus Creator3 : BusCreator  Inputs=2
  interpolation_period_m1 : Constant  Value=10
  mode_m1 : Constant  Value=8
  receive_PDO2_m1 : Subsystem
  wires:
  Bus Creator3/1 -> receive_PDO2_m1/1(mode)
  mode_m1/1 -> Bus Creator3/1  "mode_m1"
  interpolation_period_m1/1 -> Bus Creator3/2  "interpolation_period_m1"

== system ExoskeletonControlModel/DataProcessing/Working_Chart/Transparency.SetCSPforALL.ST1_set_CSP_M4 ==
  note: MOTOR 1 - MODE & INTERPOLATION TIME PERIOD
  Action Port : ActionPort
      settings: CopyFcn=Stateflow.SLINSF.SimulinkMan.removeBlockPreDeleteFcn  PreDeleteFcn=Stateflow.SLINSF.SimulinkMan.unsafePredeleteFcn
  Bus Creator3 : BusCreator  Inputs=2
  interpolation_period_m1 : Constant  Value=10
  mode_m1 : Constant  Value=8
  receive_PDO2_m1 : Subsystem
  wires:
  Bus Creator3/1 -> receive_PDO2_m1/1(mode)
  mode_m1/1 -> Bus Creator3/1  "mode_m1"
  interpolation_period_m1/1 -> Bus Creator3/2  "interpolation_period_m1"

== system ExoskeletonControlModel/DataProcessing/Working_Chart/Transparency.SetCSPforALL.ST1_set_CSP_M6 ==
  note: MOTOR 1 - MODE & INTERPOLATION TIME PERIOD
  Action Port : ActionPort
      settings: CopyFcn=Stateflow.SLINSF.SimulinkMan.removeBlockPreDeleteFcn  PreDeleteFcn=Stateflow.SLINSF.SimulinkMan.unsafePredeleteFcn
  Bus Creator3 : BusCreator  Inputs=2
  interpolation_period_m1 : Constant  Value=2
  mode_m1 : Constant  Value=8
  receive_PDO2_m1 : Subsystem
  wires:
  Bus Creator3/1 -> receive_PDO2_m1/1(mode)
  mode_m1/1 -> Bus Creator3/1  "mode_m1"
  interpolation_period_m1/1 -> Bus Creator3/2  "interpolation_period_m1"

== system ExoskeletonControlModel/DataProcessing/Working_Chart/Transparency.SetCSPforALL.ST1_set_CST_M5 ==
  note: MOTOR 1 - MODE & INTERPOLATION TIME PERIOD
  Action Port : ActionPort
      settings: CopyFcn=Stateflow.SLINSF.SimulinkMan.removeBlockPreDeleteFcn  PreDeleteFcn=Stateflow.SLINSF.SimulinkMan.unsafePredeleteFcn
  Bus Creator3 : BusCreator  Inputs=2
  interpolation_period_m1 : Constant  Value=2
  mode_m1 : Constant  Value=8
  receive_PDO2_m1 : Subsystem
  wires:
  Bus Creator3/1 -> receive_PDO2_m1/1(mode)
  mode_m1/1 -> Bus Creator3/1  "mode_m1"
  interpolation_period_m1/1 -> Bus Creator3/2  "interpolation_period_m1"

== system ExoskeletonControlModel/DataProcessing/Working_Chart/Transparency.Set_CST_M5_ShoulderFlexion.ST1_set_CST_M5 ==
  note: MOTOR 1 - MODE & INTERPOLATION TIME PERIOD
  Action Port : ActionPort
      settings: CopyFcn=Stateflow.SLINSF.SimulinkMan.removeBlockPreDeleteFcn  PreDeleteFcn=Stateflow.SLINSF.SimulinkMan.unsafePredeleteFcn
  Bus Creator3 : BusCreator  Inputs=2
  interpolation_period_m1 : Constant  Value=10
  mode_m1 : Constant  Value=10
  receive_PDO2_m1 : Subsystem
  wires:
  Bus Creator3/1 -> receive_PDO2_m1/1(mode)
  mode_m1/1 -> Bus Creator3/1  "mode_m1"
  interpolation_period_m1/1 -> Bus Creator3/2  "interpolation_period_m1"

== system ExoskeletonControlModel/DataProcessing/Working_Chart/Transparency.Set_CST_M5_ShoulderFlexion1.ST1_set_CST_M3 ==
  note: MOTOR 3 - MODE & INTERPOLATION TIME PERIOD
  Action Port : ActionPort
      settings: CopyFcn=Stateflow.SLINSF.SimulinkMan.removeBlockPreDeleteFcn  PreDeleteFcn=Stateflow.SLINSF.SimulinkMan.unsafePredeleteFcn
  Bus Creator3 : BusCreator  Inputs=2
  interpolation_period_m1 : Constant  Value=10
  mode_m1 : Constant  Value=10
  receive_PDO2_m1 : Subsystem
  wires:
  Bus Creator3/1 -> receive_PDO2_m1/1(mode)
  mode_m1/1 -> Bus Creator3/1  "mode_m1"
  interpolation_period_m1/1 -> Bus Creator3/2  "interpolation_period_m1"

== system ExoskeletonControlModel/DataProcessing/Working_Chart/Transparency.Set_CST_M5_ShoulderFlexion1.ST1_set_CST_M4 ==
  note: MOTOR 4 - MODE & INTERPOLATION TIME PERIOD
  Action Port : ActionPort
      settings: CopyFcn=Stateflow.SLINSF.SimulinkMan.removeBlockPreDeleteFcn  PreDeleteFcn=Stateflow.SLINSF.SimulinkMan.unsafePredeleteFcn
  Bus Creator3 : BusCreator  Inputs=2
  interpolation_period_m1 : Constant  Value=10
  mode_m1 : Constant  Value=10
  receive_PDO2_m1 : Subsystem
  wires:
  Bus Creator3/1 -> receive_PDO2_m1/1(mode)
  mode_m1/1 -> Bus Creator3/1  "mode_m1"
  interpolation_period_m1/1 -> Bus Creator3/2  "interpolation_period_m1"

== system ExoskeletonControlModel/DataProcessing/Working_Chart/Transparency.Set_CST_M5_ShoulderFlexion1.ST1_set_CST_M5 ==
  note: MOTOR 5 - MODE & INTERPOLATION TIME PERIOD
  Action Port : ActionPort
      settings: CopyFcn=Stateflow.SLINSF.SimulinkMan.removeBlockPreDeleteFcn  PreDeleteFcn=Stateflow.SLINSF.SimulinkMan.unsafePredeleteFcn
  Bus Creator3 : BusCreator  Inputs=2
  interpolation_period_m1 : Constant  Value=10
  mode_m1 : Constant  Value=10
  receive_PDO2_m1 : Subsystem
  wires:
  Bus Creator3/1 -> receive_PDO2_m1/1(mode)
  mode_m1/1 -> Bus Creator3/1  "mode_m1"
  interpolation_period_m1/1 -> Bus Creator3/2  "interpolation_period_m1"

== system ExoskeletonControlModel/DataProcessing/Working_Chart/Transparency.Set_CST_M6_ElbowFlexion.ST1_set_CST_M6 ==
  note: MOTOR 1 - MODE & INTERPOLATION TIME PERIOD
  Action Port : ActionPort
      settings: CopyFcn=Stateflow.SLINSF.SimulinkMan.removeBlockPreDeleteFcn  PreDeleteFcn=Stateflow.SLINSF.SimulinkMan.unsafePredeleteFcn
  Bus Creator3 : BusCreator  Inputs=2
  interpolation_period_m1 : Constant  Value=10
  mode_m1 : Constant  Value=10
  receive_PDO2_m1 : Subsystem
  wires:
  Bus Creator3/1 -> receive_PDO2_m1/1(mode)
  mode_m1/1 -> Bus Creator3/1  "mode_m1"
  interpolation_period_m1/1 -> Bus Creator3/2  "interpolation_period_m1"

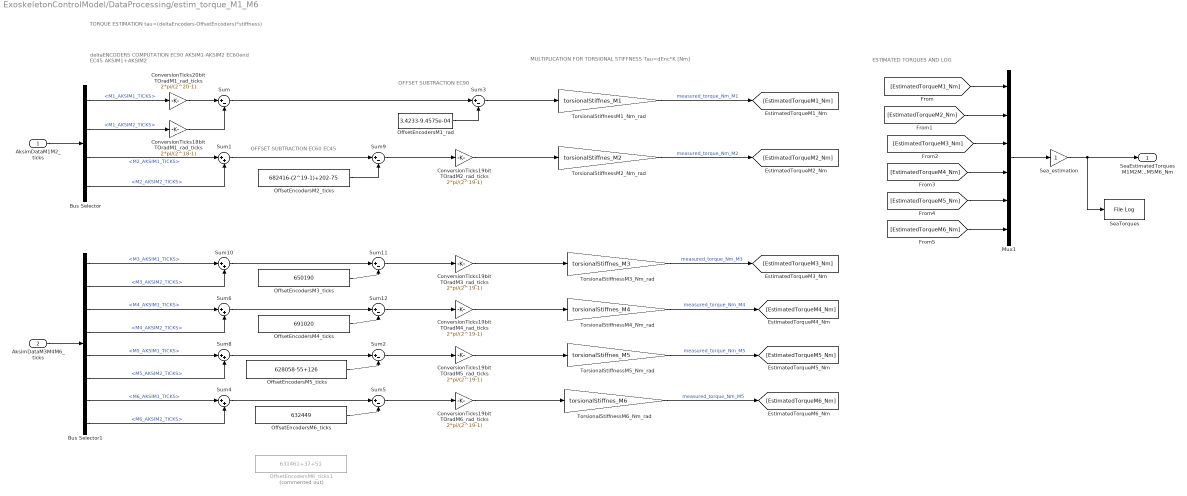
== system ExoskeletonControlModel/DataProcessing/estim_torque_M1_M6 ==
  note: ESTIMATED TORQUES AND LOG
  note: MULTIPLICATION FOR TORSIONAL STIFFNESS
      | Tau=dEnc*K [Nm]
  note: deltaENCODERS COMPUTATION
      | EC90 AKSIM1-AKSIM2
      | EC60end EC45 AKSIM1+AKSIM2
  note: OFFSET SUBTRACTION EC90
  note: OFFSET SUBTRACTION EC60 EC45
  note: TORQUE ESTIMATION tau=(deltaEncoders-OffsetEncoders)*stiffness)
  AksimDataM1M2_ticks : Inport
  AksimDataM3M4M6_ticks : Inport  Port=2
  Bus Selector : BusSelector  OutputSignals=M1_TICKS.M1_AKSIM1_TICKS,M1_TICKS.M1_AKSIM2_TICKS,M2_TICKS.M2_AKSIM1_TICKS,M2_TICKS.M2_AKSIM2_TICKS
  Bus Selector1 : BusSelector  OutputSignals=M3_TICKS.M3_AKSIM1_TICKS,M3_TICKS.M3_AKSIM2_TICKS,M4_TICKS.M4_AKSIM1_TICKS,M4_TICKS.M4_AKSIM2_TICKS,M5_TICKS.M5_AKSIM1_TICKS,M5_TICKS.M5_AKSIM2_TICKS,M6_TICKS.M6_AKSIM1_TICKS,M6_TICKS.M6_AKSIM2_TICKS
  ConversionTicks18bitTOradM1_rad_ticks : Gain  Gain=2*pi/(2^18-1)
  "ConversionTicks19bitTOradM2_rad_ticks " : Gain  Gain=2*pi/(2^19-1)
  ConversionTicks19bitTOradM3_rad_ticks : Gain  Gain=2*pi/(2^19-1)
  ConversionTicks19bitTOradM4_rad_ticks : Gain  Gain=2*pi/(2^19-1)
  ConversionTicks19bitTOradM5_rad_ticks : Gain  Gain=2*pi/(2^19-1)
  ConversionTicks19bitTOradM6_rad_ticks : Gain  Gain=2*pi/(2^19-1)
  ConversionTicks20bitTOradM1_rad_ticks : Gain  Gain=2*pi/(2^20-1)
  Mux1 : Mux  Inputs=6
  OffsetEncodersM1_rad : Constant  Value=3.4233-9.4575e-04
  OffsetEncodersM2_ticks : Constant  Value=682416-(2^19-1)+202-75
  OffsetEncodersM3_ticks : Constant  Value=650190
  OffsetEncodersM4_ticks : Constant  Value=691020
  OffsetEncodersM5_ticks : Constant  Value=628058-55+126
  OffsetEncodersM6_ticks : Constant  Value=632449
  OffsetEncodersM6_ticks1 : Constant  Commented=on  Value=631461+37+51
  SeaTorques : slrealtimeloglib/File Log  decimation=1  inputProcessing=Elements as channels (sample based)
  Sea_estimation : Gain
  Sum{,2..3,5,9,11..12} (7 alike) : Sum  Inputs=|+-
  Sum{1,4,6,8,10} (5 alike) : Sum  Inputs=|++
  TorsionalStiffnessM1_Nm_rad : Gain  Gain=torsionalStiffnes_M1  SampleTime=Ts
  TorsionalStiffnessM2_Nm_rad : Gain  Gain=torsionalStiffnes_M2
  TorsionalStiffnessM3_Nm_rad : Gain  Gain=torsionalStiffnes_M3
  TorsionalStiffnessM4_Nm_rad : Gain  Gain=torsionalStiffnes_M4
  TorsionalStiffnessM5_Nm_rad : Gain  Gain=torsionalStiffnes_M5
  TorsionalStiffnessM6_Nm_rad : Gain  Gain=torsionalStiffnes_M6
  SeaEstimatedTorquesM1M2M3M4M5M6_Nm : Outport
  wires:
  AksimDataM1M2_ticks/1 -> Bus Selector/1
  Bus Selector/1 -> ConversionTicks20bitTOradM1_rad_ticks/1  "<M1_AKSIM1_TICKS>"
  Bus Selector/2 -> ConversionTicks18bitTOradM1_rad_ticks/1  "<M1_AKSIM2_TICKS>"
  Sum/1 -> Sum3/1
  TorsionalStiffnessM1_Nm_rad/1 -> [EstimatedTorqueM1_Nm]  "measured_torque_Nm_M1"
  TorsionalStiffnessM2_Nm_rad/1 -> [EstimatedTorqueM2_Nm]  "measured_torque_Nm_M2"
  Bus Selector1/6 -> Sum8/2  "<M5_AKSIM2_TICKS>"
  TorsionalStiffnessM5_Nm_rad/1 -> [EstimatedTorqueM5_Nm]  "measured_torque_Nm_M5"
  Bus Selector1/4 -> Sum6/2  "<M4_AKSIM2_TICKS>"
  TorsionalStiffnessM3_Nm_rad/1 -> [EstimatedTorqueM3_Nm]  "measured_torque_Nm_M3"
  TorsionalStiffnessM4_Nm_rad/1 -> [EstimatedTorqueM4_Nm]  "measured_torque_Nm_M4"
  Bus Selector1/2 -> Sum10/2  "<M3_AKSIM2_TICKS>"
  ConversionTicks19bitTOradM3_rad_ticks/1 -> TorsionalStiffnessM3_Nm_rad/1
  Bus Selector1/5 -> Sum8/1  "<M5_AKSIM1_TICKS>"
  AksimDataM3M4M6_ticks/1 -> Bus Selector1/1
  Sum2/1 -> ConversionTicks19bitTOradM5_rad_ticks/1
  OffsetEncodersM5_ticks/1 -> Sum2/2
  OffsetEncodersM4_ticks/1 -> Sum12/2
  OffsetEncodersM3_ticks/1 -> Sum11/2
  "ConversionTicks19bitTOradM2_rad_ticks "/1 -> TorsionalStiffnessM2_Nm_rad/1
  Bus Selector/3 -> Sum1/1  "<M2_AKSIM1_TICKS>"
  Bus Selector/4 -> Sum1/2  "<M2_AKSIM2_TICKS>"
  Sum1/1 -> Sum9/1
  OffsetEncodersM2_ticks/1 -> Sum9/2
  Sum9/1 -> "ConversionTicks19bitTOradM2_rad_ticks "/1
  Bus Selector1/1 -> Sum10/1  "<M3_AKSIM1_TICKS>"
  Sum10/1 -> Sum11/1
  Bus Selector1/3 -> Sum6/1  "<M4_AKSIM1_TICKS>"
  Sum6/1 -> Sum12/1
  Sum12/1 -> ConversionTicks19bitTOradM4_rad_ticks/1
  ConversionTicks19bitTOradM4_rad_ticks/1 -> TorsionalStiffnessM4_Nm_rad/1
  Sum8/1 -> Sum2/1
  ConversionTicks19bitTOradM5_rad_ticks/1 -> TorsionalStiffnessM5_Nm_rad/1
  Sum11/1 -> ConversionTicks19bitTOradM3_rad_ticks/1
  Sum3/1 -> TorsionalStiffnessM1_Nm_rad/1
  OffsetEncodersM1_rad/1 -> Sum3/2
  ConversionTicks18bitTOradM1_rad_ticks/1 -> Sum/2
  ConversionTicks20bitTOradM1_rad_ticks/1 -> Sum/1
  [EstimatedTorqueM1_Nm] -> Mux1/1
  [EstimatedTorqueM2_Nm] -> Mux1/2
  [EstimatedTorqueM3_Nm] -> Mux1/3
  [EstimatedTorqueM4_Nm] -> Mux1/4
  [EstimatedTorqueM5_Nm] -> Mux1/5
  Mux1/1 -> Sea_estimation/1
  [EstimatedTorqueM6_Nm] -> Mux1/6
  Bus Selector1/7 -> Sum4/1  "<M6_AKSIM1_TICKS>"
  Bus Selector1/8 -> Sum4/2  "<M6_AKSIM2_TICKS>"
  Sum4/1 -> Sum5/1
  OffsetEncodersM6_ticks/1 -> Sum5/2
  Sum5/1 -> ConversionTicks19bitTOradM6_rad_ticks/1
  ConversionTicks19bitTOradM6_rad_ticks/1 -> TorsionalStiffnessM6_Nm_rad/1
  TorsionalStiffnessM6_Nm_rad/1 -> [EstimatedTorqueM6_Nm]  "measured_torque_Nm_M5"
  Sea_estimation/1 -> SeaTorques/1, SeaEstimatedTorquesM1M2M3M4M5M6_Nm/1

== system ExoskeletonControlModel/InputDataRX/CAN Read Loop - Channel 1 - M1-M2 ==
  note: AKSIM DATA WITHOUT DISCONTINUITIES
  note: NOTATION:
      | AKSIM_1 - BEFORE THE SPRING, IN GUI, SHORT WIRE HARDWARE, GREEN ATTACH
      | AKSIM_2 - AFTER THE SPRING, OUT GUI, LONG WIRE HARDWARE, RED ATTACH
  note: CAN MSG UNPACK
      | RECEIVE ASKIM 1 AND AKSIM 2 FROM ENCODERS
  SampleTime : Inport
  ACK : canmsglib/CAN Unpack  MsgList=(none)  MsgName=CAN Msg  MsgIDType=Standard (11-bit identifier)  MsgIdentifier=hex2dec('10C')  MsgLength=8  SignalInfo={ 'Signal1', '0', '8', 'LE', 'signed', 'Standard', '0', '1', '0', '-Inf', 'Inf' }  IDPort=off  TimestampPort=off  ErrorPort=off  RemotePort=off  LengthPort=off  StatusPort=on  ApplyMinMax=off
  Bus Creator : BusCreator  Inputs=2
  Bus Creator2 : BusCreator  Inputs=2
  Bus Creator7 : BusCreator  Inputs=2
  CAN Read : speedgoatlib_IO614/CAN/CAN Read  id=1  sampleTime=-1  portSelection=1  messageType=CAN  protl=IO614  ptIdx=0  isFDMod=0
  Terminator{,1,3..5} (5 alike) : Terminator
  While Iterator : WhileIterator  MaxIters=501  WhileBlockType=do-while
  pos_Aksim_M1 : canmsglib/CAN Unpack  MsgList=(none)  MsgName=CAN Msg  MsgIDType=Standard (11-bit identifier)  MsgIdentifier=hex2dec('502')  MsgLength=8  SignalInfo={ 'AKSIM_1', '0', '32', 'LE', 'unsigned', 'Standard', '0', '1', '0', '-Inf', 'Inf'; 'AKSIM_2', '32', '32', 'LE', 'unsigned', 'Standard', '0', '1', '0', '-Inf', 'Inf' }  IDPort=off  TimestampPort=off  ErrorPort=off  RemotePort=on  LengthPort=off  StatusPort=off  ApplyMinMax=off
  pos_Aksim_M2 : canmsglib/CAN Unpack  MsgList=(none)  MsgName=CAN Msg  MsgIDType=Standard (11-bit identifier)  MsgIdentifier=hex2dec('602')  MsgLength=8  SignalInfo={ 'AKSIM_1', '0', '32', 'LE', 'unsigned', 'Standard', '0', '1', '0', '-Inf', 'Inf'; 'AKSIM_2', '32', '32', 'LE', 'unsigned', 'Standard', '0', '1', '0', '-Inf', 'Inf' }  IDPort=off  TimestampPort=off  ErrorPort=off  RemotePort=on  LengthPort=off  StatusPort=off  ApplyMinMax=off
  aksim_data_M1_M2 : Outport
  wires:
  SampleTime/1 -> Terminator/1
  CAN Read/1 -> While Iterator/1
  ACK/2 -> Terminator1/1
  ACK/1 -> Terminator5/1
  pos_Aksim_M2/1 -> Bus Creator/1  "M2_AKSIM1_TICKS"
  CAN Read/2 -> pos_Aksim_M2/1, ACK/1, pos_Aksim_M1/1
  Bus Creator7/1 -> Bus Creator2/1  "M1_TICKS"
  Bus Creator2/1 -> aksim_data_M1_M2/1
  pos_Aksim_M2/3 -> Terminator3/1
  pos_Aksim_M1/3 -> Terminator4/1
  pos_Aksim_M1/2 -> Bus Creator7/2  "M1_AKSIM2_TICKS"
  pos_Aksim_M2/2 -> Bus Creator/2  "M2_AKSIM2_TICKS"
  pos_Aksim_M1/1 -> Bus Creator7/1  "M1_AKSIM1_TICKS"
  Bus Creator/1 -> Bus Creator2/2  "M2_TICKS"
